simulink model "AeroTabularize"  (R2024b)
settings: Solver=VariableStepAuto  StartTime=0.0  StopTime=20  RelTol=1e-3
undefined symbols (not defined in the file or in its folder): uavParam
libraries: sharedutil x4, aerolibadyn x3, aerolibtransform2 x2, matrix_library x1, aerolibatmos2 x1, aerolibutil x1
(part 1 of 2)
settings Model: Creator=mhcho  LastModifiedBy=mhcho

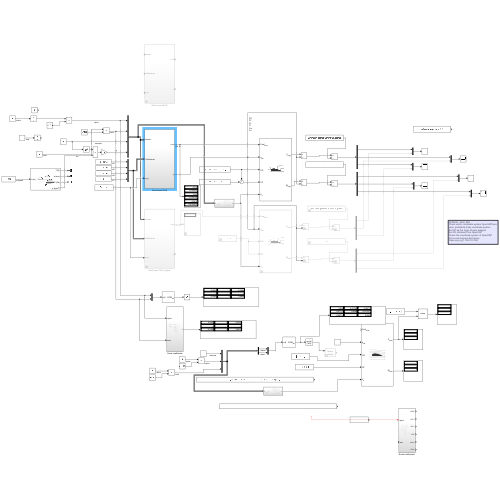
[thumbnail: Simulink's stored preview of the top-level diagram]
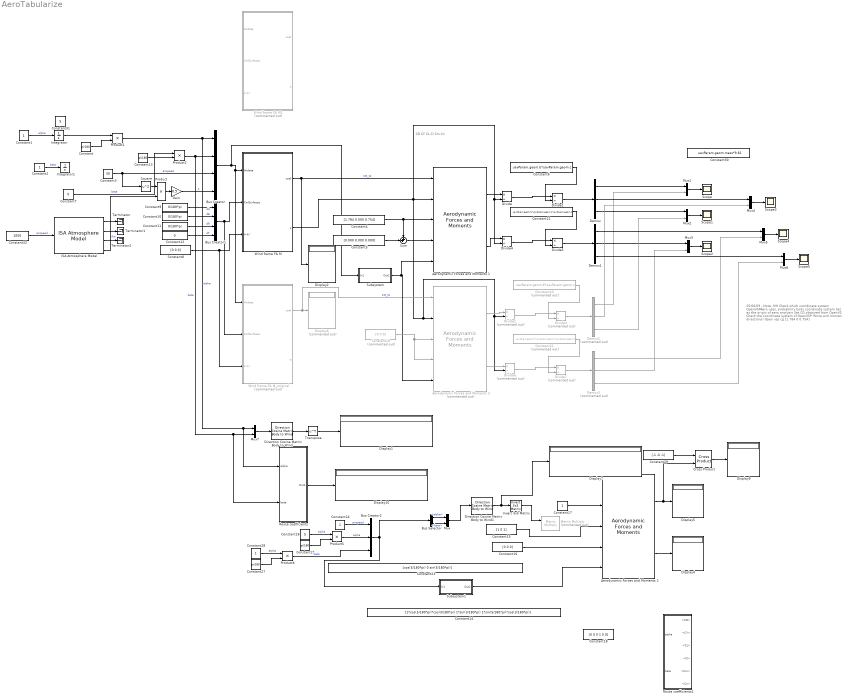
== system AeroTabularize ==
  note: CD
      | CY
      | CL
      | Cl
      | Cm
      | Cn
  note: 25/06/09 - Note, MH
      | Check which coordinate system OpenVSPAero
      | uses, probability body coordinate system
      | Set CP as the origin of aero analysis
      | Set CG obtained from OpenVSP
      | Check the coordinate system of OpenVSP
      | (force and moment directions)
      | Open vsp cg [1.784 0 0.754]
  Aerodynamic Forces and Moments 1 : aerolibadyn/Aerodynamic Forces and Moments   inputAxes=Wind  outputForceAxes=Body  outputMomentAxes=Body  S=uavParam.geom.b*uavParam.geom.c  b=uavParam.geom.b  cbar=uavParam.geom.c
  Aerodynamic Forces and Moments 2 : aerolibadyn/Aerodynamic Forces and Moments   inputAxes=Wind  outputForceAxes=Body  outputMomentAxes=Body  S=1  b=1  cbar=1
  Aerodynamic Forces and Moments 3 : aerolibadyn/Aerodynamic Forces and Moments   Commented=on  inputAxes=Wind  outputForceAxes=Body  outputMomentAxes=Body  S=uavParam.geom.b*uavParam.geom.c  b=uavParam.geom.b  cbar=uavParam.geom.c
  Bus Creator : BusCreator  Inputs=4
  Bus Creator1 : BusCreator  Inputs=4
  Bus Creator2 : BusCreator  Inputs=3
  Bus Selector : BusSelector  OutputSignals=alpha,beta
  Constant{,13,25,27} (4 alike) : Constant  Value=pi/180
  Constant{1..2,17,24,28} (5 alike) : Constant
  Constant10 : Constant  Value=0/180*pi
  Constant11 : Constant  Value=0/180*pi
  Constant12 : Constant  Value=0
  Constant14 : Constant  Value=[1*cos(5/180*pi)*cos(3/180*pi) 1*sin(3/180*pi) 1*sin(5/180*pi)*cos(3/180*pi)]
  Constant15 : Constant  Value=[1 0 1]
  Constant16 : Constant  Value=[0 0 0]
  Constant18 : Constant  Value=[0 0 0 1 0 0]
  Constant19 : Constant  Commented=on  Value=[0 0 0]
  Constant20 : Constant  Commented=on  Value=uavParam.geom.b*uavParam.geom.c
  Constant21 : Constant  Value=uavParam.geom.b*uavParam.geom.c*uavParam.geom.c
  Constant22 : Constant  Commented=on  Value=uavParam.geom.b*uavParam.geom.c*uavParam.geom.c
  Constant23 : Constant  Value=[cos(5/180*pi) 0 sin(5/180*pi)]
  Constant26 : Constant  Value=5
  Constant29 : Constant  Value=[-1 -0 -1]
  Constant3 : Constant  Value=30
  Constant30 : Constant  Value=uavParam.geom.mass*9.81
  Constant31 : Constant  Value=5
  Constant32 : Constant  Value=1000
  Constant4 : Constant  Value=[1.784 0.000 0.754]
  Constant5 : Constant  Value=[0.000 0.000 0.000]
  Constant6 : Constant  Value=uavParam.geom.b*uavParam.geom.c
  Constant7 : Constant  Value=0
  Constant8 : Constant  Value=[0 0 0]
  Constant9 : Constant  Value=0/180*pi
  Cross Product : matrix_library/Cross Product
  Demux : Demux  Outputs=3
  Demux1 : Demux  Outputs=3
  Demux2 : Demux  Commented=on  Outputs=3
  Demux3 : Demux  Commented=on  Outputs=3
  Direction Cosine Matrix Body to Wind : aerolibtransform2/Direction Cosine Matrix Body to Wind
  Direction Cosine Matrix Body to Wind1 : aerolibtransform2/Direction Cosine Matrix Body to Wind
  Display{1..2,4..5,7,9..10} (7 alike) : Display
  Display6 : Display  Commented=on
  Divide{,1,4..5} (4 alike) : Product  Inputs=*/
  Divide{2..3,6..7} (4 alike) : Product  Commented=on  Inputs=*/
  Gain : Gain  Gain=0.5
  ISA Atmosphere Model : aerolibatmos2/ISA Atmosphere Model  useExtended=off  action=Warning  custom=off  viscosityOut=off  g=9.80665  gamma=1.4  R=287.0531  L=0.0065  h_trop=11000  h_strat=20000  rho0=1.225  P0=101325  T0=288.15  h0=0  S=110.4  Tref=273.15  muref=1.716e-5
  Integrator : Integrator  InitialCondition=-5
  Integrator1 : Integrator  InitialCondition=-10
  Invert 3x3 Matrix : aerolibutil/Invert  3x3 Matrix
  Matrix Multiply : Product  Commented=on  Multiplication=Matrix(*)
  Mux{,1..7} (8 alike) : Mux  Inputs=2
  Product{,1..2,5..6} (5 alike) : Product
  Route coefficients : Subsystem
  Route coefficients1 : Subsystem
  Scope{,1..5} (6 alike) : Scope
  Square : Math  Operator=square
  Subsystem : Subsystem
  Subsystem1 : Subsystem
  Sum : Sum  Inputs=++|
  Terminator : Terminator
  Terminator1 : Terminator
  Terminator2 : Terminator
  Transpose : Math  Operator=transpose  SignedPower=on
  Wind frame F& M : Subsystem
  Wind frame F& M1 : Subsystem  Commented=on
  Wind frame F& M_original : Subsystem  Commented=on
  wires:
  Bus Creator/1 -> Subsystem/1(In1), Wind frame F& M_original/1(Airdata), Wind frame F& M/1(Airdata)
  Wind frame F& M/1(coef) -> Display2/1, Aerodynamic Forces and Moments 1/1  "FM_W"
  Wind frame F& M/2(q) -> Divide6/2, Divide2/2, Aerodynamic Forces and Moments 3/2, Aerodynamic Forces and Moments 1/2, Divide4/2, Divide/2
  Constant3/1 -> Square/1, Bus Creator/3  "airspeed"
  Gain/1 -> Bus Creator/4  "q"
  ISA Atmosphere Model/4 -> Product/2  "rho"
  Bus Creator1/1 -> Wind frame F& M_original/2(CtrlSurfaces), Wind frame F& M/2(CtrlSurfaces)
  Constant8/1 -> Wind frame F& M_original/3(p,q,r), Wind frame F& M/3(p,q,r)
  Square/1 -> Product/1
  Product/1 -> Gain/1
  Constant/1 -> Product1/2
  Constant13/1 -> Product2/2
  Product1/1 -> Route coefficients/1(alpha), Mux7/1, Bus Creator/1  "alpha"
  Product2/1 -> Route coefficients/2(beta), Mux7/2, Bus Creator/2  "beta"
  Constant16/1 -> Aerodynamic Forces and Moments 2/4
  Constant17/1 -> Aerodynamic Forces and Moments 2/2
  Aerodynamic Forces and Moments 2/2 -> Display4/1
  Aerodynamic Forces and Moments 2/1 -> Cross Product/2, Display5/1
  Wind frame F& M_original/1(coef) -> Aerodynamic Forces and Moments 3/1, Display6/1  "FM_W"
  Subsystem/1(Out1) -> Aerodynamic Forces and Moments 1/5, Aerodynamic Forces and Moments 3/5
  Constant9/1 -> Bus Creator1/1  "dA"
  Constant10/1 -> Bus Creator1/2  "dE"
  Constant11/1 -> Bus Creator1/3  "dR"
  Constant12/1 -> Bus Creator1/4  "dT"
  Aerodynamic Forces and Moments 1/1 -> Divide/1
  Divide1/1 -> Demux/1
  Divide/1 -> Divide1/1
  Constant6/1 -> Divide1/2
  Constant19/1 -> Aerodynamic Forces and Moments 3/4, Aerodynamic Forces and Moments 3/3
  Divide3/1 -> Demux2/1
  Divide2/1 -> Divide3/1
  Constant20/1 -> Divide3/2
  Aerodynamic Forces and Moments 3/1 -> Divide2/1
  Divide5/1 -> Demux1/1
  Divide4/1 -> Divide5/1
  Constant21/1 -> Divide5/2
  Aerodynamic Forces and Moments 1/2 -> Divide4/1
  Constant22/1 -> Divide7/2
  Divide7/1 -> Demux3/1
  Divide6/1 -> Divide7/1
  Aerodynamic Forces and Moments 3/2 -> Divide6/1
  Direction Cosine Matrix Body to Wind1/1 -> Display7/1, Invert 3x3 Matrix/1
  Invert 3x3 Matrix/1 -> Matrix Multiply/1
  Constant25/1 -> Product5/2
  Constant26/1 -> Product5/1  "alpha"
  Product5/1 -> Bus Creator2/2  "alpha"
  Constant27/1 -> Product6/2
  Constant28/1 -> Product6/1  "alpha"
  Product6/1 -> Bus Creator2/3  "beta"
  Constant24/1 -> Bus Creator2/1  "airspeed"
  Bus Creator2/1 -> Subsystem1/1(In1), Bus Selector/1
  Subsystem1/1(Out1) -> Aerodynamic Forces and Moments 2/5
  Bus Selector/1 -> Mux/1  "<alpha>"
  Bus Selector/2 -> Mux/2  "<beta>"
  Mux/1 -> Direction Cosine Matrix Body to Wind1/1
  Constant15/1 -> Aerodynamic Forces and Moments 2/3
  Constant29/1 -> Cross Product/1
  Cross Product/1 -> Display9/1
  Route coefficients/1(Out1) -> Display10/1
  ? -> Route coefficients1/1(alpha)
  Constant4/1 -> Sum/1, Aerodynamic Forces and Moments 1/3
  Sum/1 -> Aerodynamic Forces and Moments 1/4
  Constant5/1 -> Sum/2
  Constant1/1 -> Integrator/1  "alpha"
  Demux/1 -> Mux1/1
  Demux2/1 -> Mux1/2
  Demux/3 -> Mux2/1
  Demux1/2 -> Mux3/1
  Demux3/2 -> Mux3/2
  Mux2/1 -> Scope1/1
  Mux3/1 -> Scope2/1
  Mux1/1 -> Scope/1
  Demux2/3 -> Mux2/2
  Mux4/1 -> Scope3/1
  Demux/2 -> Mux4/1
  Demux2/2 -> Mux4/2
  Mux5/1 -> Scope4/1
  Demux1/1 -> Mux5/1
  Demux3/1 -> Mux5/2
  Mux6/1 -> Scope5/1
  Demux1/3 -> Mux6/1
  Demux3/3 -> Mux6/2
  Constant2/1 -> Integrator1/1  "beta"
  Direction Cosine Matrix Body to Wind/1 -> Transpose/1
  Mux7/1 -> Direction Cosine Matrix Body to Wind/1
  Transpose/1 -> Display1/1
  Constant32/1 -> ISA Atmosphere Model/1  "airspeed"
  ISA Atmosphere Model/1 -> Terminator/1
  ISA Atmosphere Model/2 -> Terminator1/1
  ISA Atmosphere Model/3 -> Terminator2/1
  Constant7/1 -> Product2/1  "beta"
  Integrator/1 -> Product1/1

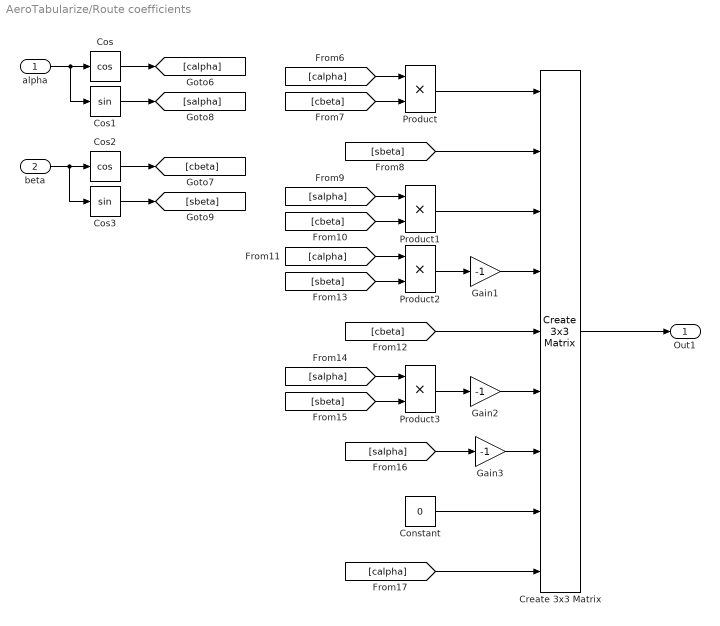
== system AeroTabularize/Route coefficients ==
  alpha : Inport
  beta : Inport  Port=2
  Constant : Constant  Value=0
  Cos : Trigonometry  Operator=cos
  Cos1 : Trigonometry
  Cos2 : Trigonometry  Operator=cos
  Cos3 : Trigonometry
  Create 3x3 Matrix : sharedutil/Create 3x3 Matrix  aMode=aMode
  Gain1 : Gain  Gain=-1
  Gain2 : Gain  Gain=-1
  Gain3 : Gain  Gain=-1
  Product{,1..3} (4 alike) : Product
  Out1 : Outport
  wires:
  Cos/1 -> [calpha]
  alpha/1 -> Cos1/1, Cos/1
  Cos1/1 -> [salpha]
  Cos2/1 -> [cbeta]
  Cos3/1 -> [sbeta]
  beta/1 -> Cos3/1, Cos2/1
  [calpha] -> Product/1
  [cbeta] -> Product/2
  Product/1 -> Create 3x3 Matrix/1
  [sbeta] -> Create 3x3 Matrix/2
  Product1/1 -> Create 3x3 Matrix/3
  [salpha] -> Product1/1
  [cbeta] -> Product1/2
  [calpha] -> Product2/1
  Product2/1 -> Gain1/1
  [sbeta] -> Product2/2
  Gain1/1 -> Create 3x3 Matrix/4
  [cbeta] -> Create 3x3 Matrix/5
  Product3/1 -> Gain2/1
  [salpha] -> Product3/1
  [sbeta] -> Product3/2
  Gain2/1 -> Create 3x3 Matrix/6
  Gain3/1 -> Create 3x3 Matrix/7
  [salpha] -> Gain3/1
  Constant/1 -> Create 3x3 Matrix/8
  [calpha] -> Create 3x3 Matrix/9
  Create 3x3 Matrix/1 -> Out1/1

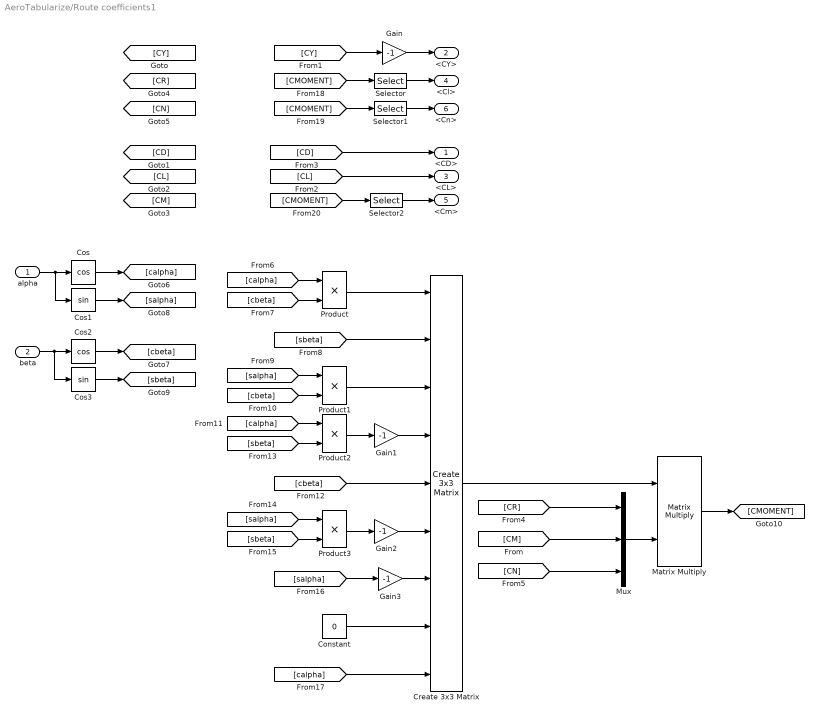
== system AeroTabularize/Route coefficients1 ==
  alpha : Inport
  beta : Inport  Port=2
  Constant : Constant  Value=0
  Cos : Trigonometry  Operator=cos
  Cos1 : Trigonometry
  Cos2 : Trigonometry  Operator=cos
  Cos3 : Trigonometry
  Create 3x3 Matrix : sharedutil/Create 3x3 Matrix  aMode=aMode
  Gain{,1..3} (4 alike) : Gain  Gain=-1
  Matrix Multiply : Product  Multiplication=Matrix(*)
  Mux : Mux  Inputs=3
  Product{,1..3} (4 alike) : Product
  Selector : Selector  InputPortWidth=3  IndexOptions=Index vector (dialog)  Indices=[1]  OutputSizes=1
  Selector1 : Selector  InputPortWidth=3  IndexOptions=Index vector (dialog)  Indices=[3]  OutputSizes=1
  Selector2 : Selector  InputPortWidth=3  IndexOptions=Index vector (dialog)  Indices=[2]  OutputSizes=1
  <CD> : Outport
  <CY> : Outport  Port=2
  <CL> : Outport  Port=3
  <Cl> : Outport  Port=4
  <Cm> : Outport  Port=5
  <Cn> : Outport  Port=6
  wires:
  ? -> [CY]
  [CY] -> Gain/1
  ? -> [CD]
  ? -> [CL]
  [CL] -> <CL>/1
  [CD] -> <CD>/1
  ? -> [CM]
  ? -> [CR]
  ? -> [CN]
  Gain/1 -> <CY>/1
  Cos/1 -> [calpha]
  alpha/1 -> Cos1/1, Cos/1
  Cos1/1 -> [salpha]
  Cos2/1 -> [cbeta]
  Cos3/1 -> [sbeta]
  beta/1 -> Cos3/1, Cos2/1
  [calpha] -> Product/1
  [cbeta] -> Product/2
  Product/1 -> Create 3x3 Matrix/1
  [sbeta] -> Create 3x3 Matrix/2
  Product1/1 -> Create 3x3 Matrix/3
  [salpha] -> Product1/1
  [cbeta] -> Product1/2
  [calpha] -> Product2/1
  Product2/1 -> Gain1/1
  [sbeta] -> Product2/2
  Gain1/1 -> Create 3x3 Matrix/4
  [cbeta] -> Create 3x3 Matrix/5
  Product3/1 -> Gain2/1
  [salpha] -> Product3/1
  [sbeta] -> Product3/2
  Gain2/1 -> Create 3x3 Matrix/6
  Gain3/1 -> Create 3x3 Matrix/7
  [salpha] -> Gain3/1
  Constant/1 -> Create 3x3 Matrix/8
  [calpha] -> Create 3x3 Matrix/9
  Create 3x3 Matrix/1 -> Matrix Multiply/1
  Mux/1 -> Matrix Multiply/2
  [CM] -> Mux/2
  [CR] -> Mux/1
  [CN] -> Mux/3
  Matrix Multiply/1 -> [CMOMENT]
  Selector/1 -> <Cl>/1
  [CMOMENT] -> Selector/1
  Selector1/1 -> <Cn>/1
  [CMOMENT] -> Selector1/1
  [CMOMENT] -> Selector2/1
  Selector2/1 -> <Cm>/1

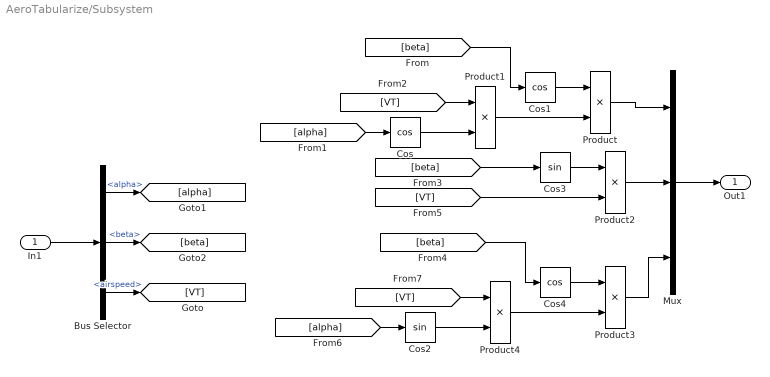
== system AeroTabularize/Subsystem ==
  In1 : Inport
  Bus Selector : BusSelector  OutputSignals=alpha,beta,airspeed
  Cos : Trigonometry  Operator=cos
  Cos1 : Trigonometry  Operator=cos
  Cos2 : Trigonometry
  Cos3 : Trigonometry
  Cos4 : Trigonometry  Operator=cos
  Mux : Mux  Inputs=3
  Product{,1..4} (5 alike) : Product
  Out1 : Outport
  wires:
  In1/1 -> Bus Selector/1
  Bus Selector/3 -> [VT]  "<airspeed>"
  Bus Selector/1 -> [alpha]  "<alpha>"
  Bus Selector/2 -> [beta]  "<beta>"
  Mux/1 -> Out1/1
  Product/1 -> Mux/1
  Product1/1 -> Product/2
  Cos/1 -> Product1/2
  Cos1/1 -> Product/1
  [alpha] -> Cos/1
  [VT] -> Product1/1
  [beta] -> Cos1/1
  Cos3/1 -> Product2/1
  [beta] -> Cos3/1
  [VT] -> Product2/2
  Product2/1 -> Mux/2
  Cos4/1 -> Product3/1
  [VT] -> Product4/1
  [alpha] -> Cos2/1
  [beta] -> Cos4/1
  Product4/1 -> Product3/2
  Cos2/1 -> Product4/2
  Product3/1 -> Mux/3

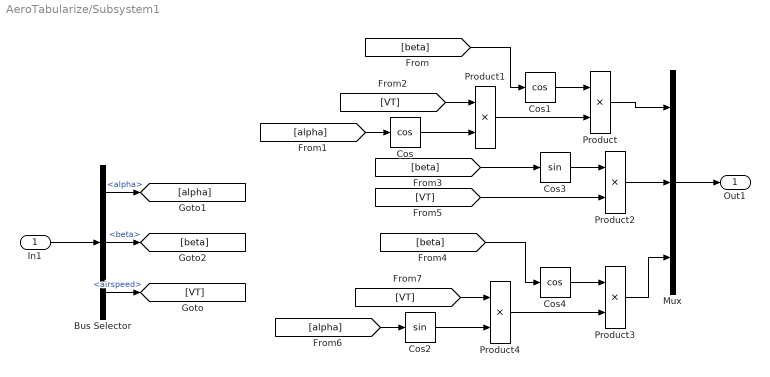
== system AeroTabularize/Subsystem1 ==
  In1 : Inport
  Bus Selector : BusSelector  OutputSignals=alpha,beta,airspeed
  Cos : Trigonometry  Operator=cos
  Cos1 : Trigonometry  Operator=cos
  Cos2 : Trigonometry
  Cos3 : Trigonometry
  Cos4 : Trigonometry  Operator=cos
  Mux : Mux  Inputs=3
  Product{,1..4} (5 alike) : Product
  Out1 : Outport
  wires:
  In1/1 -> Bus Selector/1
  Bus Selector/3 -> [VT]  "<airspeed>"
  Bus Selector/1 -> [alpha]  "<alpha>"
  Bus Selector/2 -> [beta]  "<beta>"
  Mux/1 -> Out1/1
  Product/1 -> Mux/1
  Product1/1 -> Product/2
  Cos/1 -> Product1/2
  Cos1/1 -> Product/1
  [alpha] -> Cos/1
  [VT] -> Product1/1
  [beta] -> Cos1/1
  Cos3/1 -> Product2/1
  [beta] -> Cos3/1
  [VT] -> Product2/2
  Product2/1 -> Mux/2
  Cos4/1 -> Product3/1
  [VT] -> Product4/1
  [alpha] -> Cos2/1
  [beta] -> Cos4/1
  Product4/1 -> Product3/2
  Cos2/1 -> Product4/2
  Product3/1 -> Mux/3

== system AeroTabularize/Wind frame F& M ==
  Airdata : Inport
  CtrlSurfaces : Inport  Port=2
  p,q,r : Inport  Port=3
  Bus Selector : BusSelector  OutputSignals=q
  Bus Selector1 : BusSelector  OutputSignals=dA,dR
  Bus Selector2 : BusSelector  OutputSignals=dE
  Bus Selector3 : BusSelector  OutputSignals=dA,dR
  Bus Selector4 : BusSelector  OutputSignals=alpha,beta
  Bus Selector6 : BusSelector  OutputSignals=alpha,beta,airspeed
  Bus Selector7 : BusSelector  OutputSignals=alpha,airspeed
  Lateral Channel : Subsystem
  Longitudinal Channel : Subsystem
  Mux : Mux  Inputs=6
  Route coefficients : Subsystem
  coef : Outport  PortDimensions=6  VectorParamsAs1DForOutWhenUnconnected=off
  q : Outport  Port=2
  wires:
  Bus Selector7/2 -> Longitudinal Channel/2(Airpseed)  "<airspeed>"
  Bus Selector7/1 -> Longitudinal Channel/1(alpha)  "<alpha>"
  Bus Selector6/3 -> Lateral Channel/3(Airspeed)  "<airspeed>"
  Bus Selector6/2 -> Lateral Channel/2(beta)  "<beta>"
  Airdata/1 -> Bus Selector7/1, Bus Selector6/1, Bus Selector4/1, Bus Selector/1
  Bus Selector2/1 -> Longitudinal Channel/3(dE)  "<dE>"
  Bus Selector1/2 -> Lateral Channel/5(dR)  "<dR>"
  Bus Selector1/1 -> Lateral Channel/4(dA)  "<dA>"
  CtrlSurfaces/1 -> Bus Selector3/1, Bus Selector2/1, Bus Selector1/1
  p,q,r/1 -> Lateral Channel/6(p,q,r), Longitudinal Channel/4(p,q,r)
  Mux/1 -> coef/1
  Longitudinal Channel/1(Longitudinal) -> Route coefficients/2(Longitudinal)
  Route coefficients/1(<CD>) -> Mux/1
  Route coefficients/2(<CC>) -> Mux/2
  Route coefficients/3(<CL>) -> Mux/3
  Route coefficients/4(<Cl>) -> Mux/4
  Route coefficients/5(<Cm>) -> Mux/5
  Route coefficients/6(<Cn>) -> Mux/6
  Bus Selector/1 -> q/1  "<q>"
  Bus Selector3/1 -> Longitudinal Channel/5(dA)  "<dA>"
  Bus Selector3/2 -> Longitudinal Channel/6(dR)  "<dR>"
  Lateral Channel/1(Lateral) -> Route coefficients/1(Lateral)
  Bus Selector4/1 -> Route coefficients/3(alpha)  "<alpha>"
  Bus Selector4/2 -> Route coefficients/4(beta)  "<beta>"
  Bus Selector6/1 -> Lateral Channel/1(alpha)  "<alpha>"

== system AeroTabularize/Wind frame F& M1 ==
  Airdata : Inport
  CtrlSurfaces : Inport  Port=2
  p,q,r : Inport  Port=3
  Bus Selector : BusSelector  OutputSignals=q
  Bus Selector1 : BusSelector  OutputSignals=dA,dR
  Bus Selector2 : BusSelector  OutputSignals=dE
  Bus Selector3 : BusSelector  OutputSignals=dA,dR
  Bus Selector4 : BusSelector  OutputSignals=alpha,beta
  Bus Selector6 : BusSelector  OutputSignals=beta,airspeed
  Bus Selector7 : BusSelector  OutputSignals=alpha,airspeed
  Lateral Channel : Subsystem
  Longitudinal Channel : Subsystem
  Mux : Mux  Inputs=6
  Route coefficients : Subsystem
  coef : Outport  PortDimensions=6  VectorParamsAs1DForOutWhenUnconnected=off
  q : Outport  Port=2
  wires:
  Bus Selector7/2 -> Longitudinal Channel/2(Airpseed)  "<airspeed>"
  Bus Selector7/1 -> Longitudinal Channel/1(alpha)  "<alpha>"
  Bus Selector6/2 -> Lateral Channel/2(Airspeed)  "<airspeed>"
  Bus Selector6/1 -> Lateral Channel/1(beta)  "<beta>"
  Airdata/1 -> Bus Selector4/1, Bus Selector/1, Bus Selector6/1, Bus Selector7/1
  Bus Selector2/1 -> Longitudinal Channel/3(dE)  "<dE>"
  Bus Selector1/2 -> Lateral Channel/4(dR)  "<dR>"
  Bus Selector1/1 -> Lateral Channel/3(dA)  "<dA>"
  CtrlSurfaces/1 -> Bus Selector1/1, Bus Selector3/1, Bus Selector2/1
  p,q,r/1 -> Lateral Channel/5(p,q,r), Longitudinal Channel/4(p,q,r)
  Mux/1 -> coef/1
  Longitudinal Channel/1(Longitudinal) -> Route coefficients/2(Longitudinal)
  Route coefficients/1(<CD>) -> Mux/1
  Route coefficients/2(<CY>) -> Mux/2
  Route coefficients/3(<CL>) -> Mux/3
  Route coefficients/4(<Cl>) -> Mux/4
  Route coefficients/5(<Cm>) -> Mux/5
  Route coefficients/6(<Cn>) -> Mux/6
  Bus Selector/1 -> q/1  "<q>"
  Bus Selector3/1 -> Longitudinal Channel/5(dA)  "<dA>"
  Bus Selector3/2 -> Longitudinal Channel/6(dR)  "<dR>"
  Lateral Channel/1(Lateral) -> Route coefficients/1(Lateral)
  Bus Selector4/1 -> Route coefficients/3(alpha)  "<alpha>"
  Bus Selector4/2 -> Route coefficients/4(beta)  "<beta>"

== system AeroTabularize/Wind frame F& M_original ==
  Airdata : Inport
  CtrlSurfaces : Inport  Port=2
  p,q,r : Inport  Port=3
  Bus Selector : BusSelector  OutputSignals=q
  Bus Selector1 : BusSelector  OutputSignals=dA,dR
  Bus Selector2 : BusSelector  OutputSignals=dE,dA,dR
  Bus Selector6 : BusSelector  OutputSignals=beta,airspeed
  Bus Selector7 : BusSelector  OutputSignals=alpha,airspeed
  Lateral Channel : Subsystem
  Longitudinal Channel : Subsystem
  Mux : Mux  Inputs=6
  Route coefficients : Subsystem
  coef : Outport  PortDimensions=6  VectorParamsAs1DForOutWhenUnconnected=off
  q : Outport  Port=2
  wires:
  Bus Selector7/2 -> Longitudinal Channel/2(Airpseed)  "<airspeed>"
  Bus Selector7/1 -> Longitudinal Channel/1(alpha)  "<alpha>"
  Bus Selector6/2 -> Lateral Channel/2(Airspeed)  "<airspeed>"
  Bus Selector6/1 -> Lateral Channel/1(beta)  "<beta>"
  Airdata/1 -> Bus Selector/1, Bus Selector6/1, Bus Selector7/1
  Bus Selector2/1 -> Longitudinal Channel/3(dE)  "<dE>"
  Bus Selector1/2 -> Lateral Channel/4(dR)  "<dR>"
  Bus Selector1/1 -> Lateral Channel/3(dA)  "<dA>"
  CtrlSurfaces/1 -> Bus Selector1/1, Bus Selector2/1
  p,q,r/1 -> Lateral Channel/5(p,q,r), Longitudinal Channel/4(p,q,r)
  Bus Selector2/2 -> Longitudinal Channel/5(dA)  "<dA>"
  Bus Selector2/3 -> Longitudinal Channel/6(dR)  "<dR>"
  Mux/1 -> coef/1
  Lateral Channel/1(Lateral) -> Route coefficients/1(Lateral)
  Longitudinal Channel/1(Longitudinal) -> Route coefficients/2(Longitudinal)
  Route coefficients/1(<CD>) -> Mux/1
  Route coefficients/2(<CY>) -> Mux/2
  Route coefficients/3(<CL>) -> Mux/3
  Route coefficients/4(<Cl>) -> Mux/4
  Route coefficients/5(<Cm>) -> Mux/5
  Route coefficients/6(<Cn>) -> Mux/6
  Bus Selector/1 -> q/1  "<q>"

== system AeroTabularize/Wind frame F& M/Lateral Channel ==
  alpha : Inport
  beta : Inport  Port=2
  Airspeed : Inport  Port=3
  dA : Inport  Port=4
  dR : Inport  Port=5
  p,q,r : Inport  Port=6
  Bus Creator : BusCreator  Inputs=3
  CY : Subsystem
  Cl : Subsystem
  Cn : Subsystem
  Lateral : Outport  VectorParamsAs1DForOutWhenUnconnected=off
  wires:
  p,q,r/1 -> CY/4(p,q,r), Cl/5(p,q,r), Cn/5(p,q,r)
  Airspeed/1 -> CY/5(Airspeed), Cl/6(Airspeed), Cn/6(Airspeed)
  dR/1 -> CY/3(dR), Cl/4(dR), Cn/4(dR)
  dA/1 -> Cn/3(dA), Cl/3(dA)
  beta/1 -> CY/2(beta), Cn/2(beta), Cl/2(beta)
  Bus Creator/1 -> Lateral/1
  CY/1(CS) -> Bus Creator/1  "CS"
  alpha/1 -> Cn/1(alpha), Cl/1(alpha), CY/1(alpha)
  Cl/1(Cl) -> Bus Creator/2  "Cl"
  Cn/1(Cn) -> Bus Creator/3  "Cn"

== system AeroTabularize/Wind frame F& M/Longitudinal Channel ==
  alpha : Inport
  Airpseed : Inport  Port=2
  dE : Inport  Port=3
  p,q,r : Inport  Port=4
  dA : Inport  Port=5
  dR : Inport  Port=6
  Bus Creator : BusCreator  Inputs=3
  CD : Subsystem
  CL : Subsystem
  Cm : Subsystem
  Saturation : Saturate  UpperLimit=max(uavParam.aero.alpha_lon)  LowerLimit=min(uavParam.aero.alpha_lon)  LinearizeAsGain=off  ZeroCross=off
  Transfer Fcn : TransferFcn  Numerator=[1 0]  Denominator=[0.1 1]
  Longitudinal : Outport  VectorParamsAs1DForOutWhenUnconnected=off
  wires:
  Transfer Fcn/1 -> CL/2(alpha_dot)
  Airpseed/1 -> CL/5(Airspeed), Cm/4(Airspeed)
  p,q,r/1 -> CL/4(p,q,r), Cm/3(p,q,r)
  Bus Creator/1 -> Longitudinal/1
  dE/1 -> Cm/2(dE), CD/4(dE), CL/3(dE)
  CD/1(CD) -> Bus Creator/1  "CD"
  alpha/1 -> Saturation/1
  dR/1 -> CD/3(dR)
  dA/1 -> CD/2(dA), CL/6(dA)
  Saturation/1 -> CD/1(alpha), CL/1(alpha), Cm/1(alpha), Transfer Fcn/1
  Cm/1(Cm) -> Bus Creator/3  "Cm"
  CL/1(CL) -> Bus Creator/2  "CL"

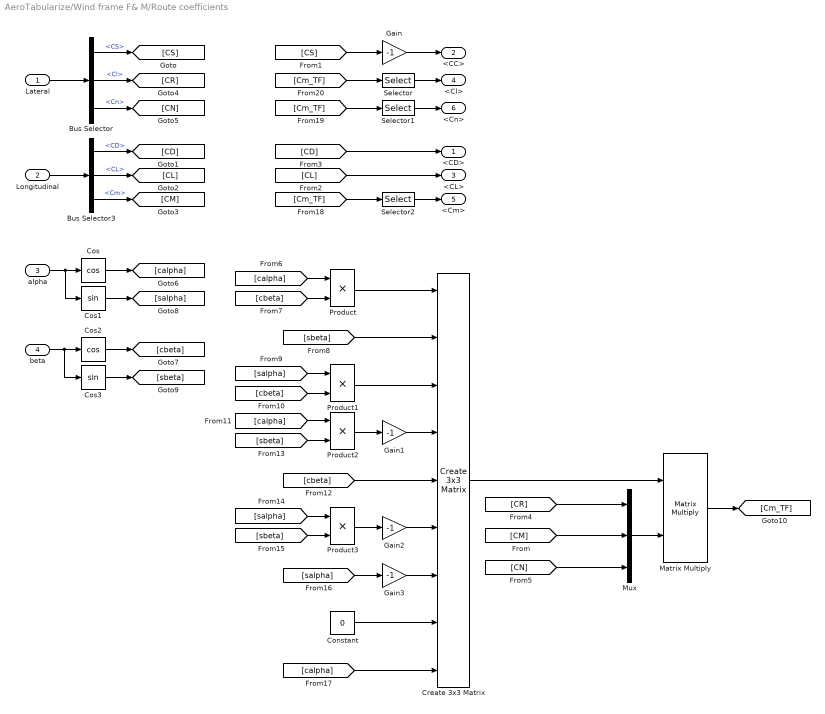
== system AeroTabularize/Wind frame F& M/Route coefficients ==
  Lateral : Inport
  Longitudinal : Inport  Port=2
  alpha : Inport  Port=3
  beta : Inport  Port=4
  Bus Selector : BusSelector  OutputSignals=CS,Cl,Cn
  Bus Selector3 : BusSelector  OutputSignals=CD,CL,Cm
  Constant : Constant  Value=0
  Cos : Trigonometry  Operator=cos
  Cos1 : Trigonometry
  Cos2 : Trigonometry  Operator=cos
  Cos3 : Trigonometry
  Create 3x3 Matrix : sharedutil/Create 3x3 Matrix  aMode=aMode
      settings: LibrarySourceBlock=aerolibutil/Create 3x3 Matrix
  Gain{,1..3} (4 alike) : Gain  Gain=-1
  Matrix Multiply : Product  Multiplication=Matrix(*)
  Mux : Mux  Inputs=3
  Product{,1..3} (4 alike) : Product
  Selector : Selector  InputPortWidth=3  IndexOptions=Index vector (dialog)  Indices=[1]  OutputSizes=1
  Selector1 : Selector  InputPortWidth=3  IndexOptions=Index vector (dialog)  Indices=[3]  OutputSizes=1
  Selector2 : Selector  InputPortWidth=3  IndexOptions=Index vector (dialog)  Indices=[2]  OutputSizes=1
  <CD> : Outport
  <CC> : Outport  Port=2
  <CL> : Outport  Port=3
  <Cl> : Outport  Port=4
  <Cm> : Outport  Port=5
  <Cn> : Outport  Port=6
  wires:
  Lateral/1 -> Bus Selector/1
  Longitudinal/1 -> Bus Selector3/1
  Bus Selector/1 -> [CS]  "<CS>"
  Bus Selector3/1 -> [CD]  "<CD>"
  Bus Selector3/2 -> [CL]  "<CL>"
  [CL] -> <CL>/1
  [CD] -> <CD>/1
  Bus Selector3/3 -> [CM]  "<Cm>"
  Bus Selector/2 -> [CR]  "<Cl>"
  Bus Selector/3 -> [CN]  "<Cn>"
  Cos/1 -> [calpha]
  alpha/1 -> Cos1/1, Cos/1
  Cos1/1 -> [salpha]
  Cos2/1 -> [cbeta]
  Cos3/1 -> [sbeta]
  beta/1 -> Cos3/1, Cos2/1
  [calpha] -> Product/1
  [cbeta] -> Product/2
  Product/1 -> Create 3x3 Matrix/1
  [sbeta] -> Create 3x3 Matrix/2
  Product1/1 -> Create 3x3 Matrix/3
  [salpha] -> Product1/1
  [cbeta] -> Product1/2
  [calpha] -> Product2/1
  Product2/1 -> Gain1/1
  [sbeta] -> Product2/2
  Gain1/1 -> Create 3x3 Matrix/4
  [cbeta] -> Create 3x3 Matrix/5
  Product3/1 -> Gain2/1
  [salpha] -> Product3/1
  [sbeta] -> Product3/2
  Gain2/1 -> Create 3x3 Matrix/6
  Gain3/1 -> Create 3x3 Matrix/7
  [salpha] -> Gain3/1
  Constant/1 -> Create 3x3 Matrix/8
  [calpha] -> Create 3x3 Matrix/9
  Create 3x3 Matrix/1 -> Matrix Multiply/1
  Mux/1 -> Matrix Multiply/2
  [CM] -> Mux/2
  Matrix Multiply/1 -> [Cm_TF]
  [Cm_TF] -> Selector/1
  [Cm_TF] -> Selector1/1
  [Cm_TF] -> Selector2/1
  [CR] -> Mux/1
  [CN] -> Mux/3
  Gain/1 -> <CC>/1
  [CS] -> Gain/1
  Selector2/1 -> <Cm>/1
  Selector/1 -> <Cl>/1
  Selector1/1 -> <Cn>/1

== system AeroTabularize/Wind frame F& M1/Lateral Channel ==
  beta : Inport
  Airspeed : Inport  Port=2
  dA : Inport  Port=3
  dR : Inport  Port=4
  p,q,r : Inport  Port=5
  Bus Creator : BusCreator  Inputs=3
  CY : Subsystem
  Cl : Subsystem
  Cn : Subsystem
  Lateral : Outport  VectorParamsAs1DForOutWhenUnconnected=off
  wires:
  p,q,r/1 -> Cn/4(p,q,r), Cl/4(p,q,r), CY/3(p,q,r)
  Airspeed/1 -> Cn/5(Airspeed), Cl/5(Airspeed), CY/4(Airspeed)
  dR/1 -> Cn/3(dR), Cl/3(dR), CY/2(dR)
  dA/1 -> Cl/2(dA), Cn/2(dA)
  beta/1 -> CY/1(beta), Cl/1(beta), Cn/1(beta)
  Bus Creator/1 -> Lateral/1
  CY/1(CY) -> Bus Creator/1  "CY"
  Cl/1(Cl) -> Bus Creator/2  "Cl"
  Cn/1(Cn) -> Bus Creator/3  "Cn"

== system AeroTabularize/Wind frame F& M1/Longitudinal Channel ==
  alpha : Inport
  Airpseed : Inport  Port=2
  dE : Inport  Port=3
  p,q,r : Inport  Port=4
  dA : Inport  Port=5
  dR : Inport  Port=6
  Bus Creator : BusCreator  Inputs=3
  CD : Subsystem
  CL : Subsystem
  Cm : Subsystem
  Saturation : Saturate  UpperLimit=max(uavParam.aero.alpha)  LowerLimit=min(uavParam.aero.alpha)  LinearizeAsGain=off  ZeroCross=off
  Transfer Fcn : TransferFcn  Numerator=[1 0]  Denominator=[0.1 1]
  Longitudinal : Outport  VectorParamsAs1DForOutWhenUnconnected=off
  wires:
  Transfer Fcn/1 -> CL/2(alpha_dot)
  Airpseed/1 -> CL/5(Airspeed), Cm/4(Airspeed)
  p,q,r/1 -> CL/4(p,q,r), Cm/3(p,q,r)
  Bus Creator/1 -> Longitudinal/1
  dE/1 -> Cm/2(dE), CD/4(dE), CL/3(dE)
  CD/1(CD) -> Bus Creator/1  "CD"
  alpha/1 -> Saturation/1
  dR/1 -> CD/3(dR)
  dA/1 -> CD/2(dA), CL/6(dA)
  Saturation/1 -> CD/1(alpha), CL/1(alpha), Cm/1(alpha), Transfer Fcn/1
  Cm/1(Cm) -> Bus Creator/3  "Cm"
  CL/1(CL) -> Bus Creator/2  "CL"

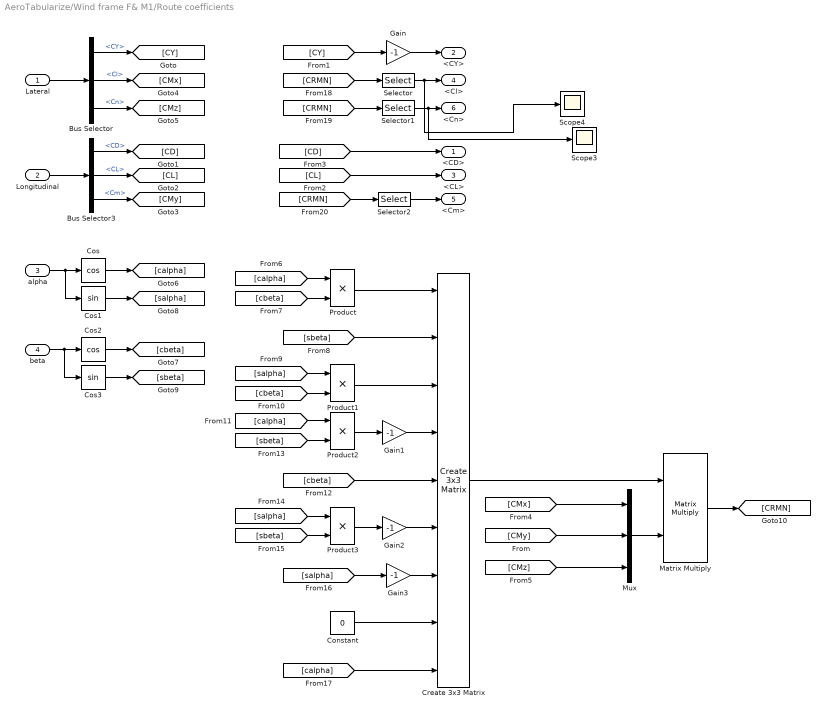
== system AeroTabularize/Wind frame F& M1/Route coefficients ==
  Lateral : Inport
  Longitudinal : Inport  Port=2
  alpha : Inport  Port=3
  beta : Inport  Port=4
  Bus Selector : BusSelector  OutputSignals=CY,Cl,Cn
  Bus Selector3 : BusSelector  OutputSignals=CD,CL,Cm
  Constant : Constant  Value=0
  Cos : Trigonometry  Operator=cos
  Cos1 : Trigonometry
  Cos2 : Trigonometry  Operator=cos
  Cos3 : Trigonometry
  Create 3x3 Matrix : sharedutil/Create 3x3 Matrix  aMode=aMode
      settings: LibrarySourceBlock=aerolibutil/Create 3x3 Matrix
  Gain{,1..3} (4 alike) : Gain  Gain=-1
  Matrix Multiply : Product  Multiplication=Matrix(*)
  Mux : Mux  Inputs=3
  Product{,1..3} (4 alike) : Product
  Scope3 : Scope
  Scope4 : Scope
  Selector : Selector  InputPortWidth=3  IndexOptions=Index vector (dialog)  Indices=[1]  OutputSizes=1
  Selector1 : Selector  InputPortWidth=3  IndexOptions=Index vector (dialog)  Indices=[3]  OutputSizes=1
  Selector2 : Selector  InputPortWidth=3  IndexOptions=Index vector (dialog)  Indices=[2]  OutputSizes=1
  <CD> : Outport
  <CY> : Outport  Port=2
  <CL> : Outport  Port=3
  <Cl> : Outport  Port=4
  <Cm> : Outport  Port=5
  <Cn> : Outport  Port=6
  wires:
  Lateral/1 -> Bus Selector/1
  Longitudinal/1 -> Bus Selector3/1
  Bus Selector/1 -> [CY]  "<CY>"
  Bus Selector3/1 -> [CD]  "<CD>"
  Bus Selector3/2 -> [CL]  "<CL>"
  [CL] -> <CL>/1
  [CD] -> <CD>/1
  Bus Selector3/3 -> [CMy]  "<Cm>"
  Bus Selector/2 -> [CMx]  "<Cl>"
  Bus Selector/3 -> [CMz]  "<Cn>"
  [CY] -> Gain/1
  Cos/1 -> [calpha]
  alpha/1 -> Cos1/1, Cos/1
  Cos1/1 -> [salpha]
  Cos2/1 -> [cbeta]
  Cos3/1 -> [sbeta]
  beta/1 -> Cos3/1, Cos2/1
  [calpha] -> Product/1
  [cbeta] -> Product/2
  Product/1 -> Create 3x3 Matrix/1
  [sbeta] -> Create 3x3 Matrix/2
  Product1/1 -> Create 3x3 Matrix/3
  [salpha] -> Product1/1
  [cbeta] -> Product1/2
  [calpha] -> Product2/1
  Product2/1 -> Gain1/1
  [sbeta] -> Product2/2
  Gain1/1 -> Create 3x3 Matrix/4
  [cbeta] -> Create 3x3 Matrix/5
  Product3/1 -> Gain2/1
  [salpha] -> Product3/1
  [sbeta] -> Product3/2
  Gain2/1 -> Create 3x3 Matrix/6
  Gain3/1 -> Create 3x3 Matrix/7
  [salpha] -> Gain3/1
  Constant/1 -> Create 3x3 Matrix/8
  [calpha] -> Create 3x3 Matrix/9
  Create 3x3 Matrix/1 -> Matrix Multiply/1
  Mux/1 -> Matrix Multiply/2
  [CMy] -> Mux/2
  Matrix Multiply/1 -> [CRMN]
  Selector/1 -> Scope4/1, <Cl>/1
  [CRMN] -> Selector/1
  Selector1/1 -> Scope3/1, <Cn>/1
  [CRMN] -> Selector1/1
  [CRMN] -> Selector2/1
  Selector2/1 -> <Cm>/1
  [CMx] -> Mux/1
  [CMz] -> Mux/3
  Gain/1 -> <CY>/1

== system AeroTabularize/Wind frame F& M_original/Lateral Channel ==
  beta : Inport
  Airspeed : Inport  Port=2
  dA : Inport  Port=3
  dR : Inport  Port=4
  p,q,r : Inport  Port=5
  Bus Creator : BusCreator  Inputs=3
  CY : Subsystem
  Cl : Subsystem
  Cn : Subsystem
  Lateral : Outport  VectorParamsAs1DForOutWhenUnconnected=off
  wires:
  Cl/1(Cl) -> Bus Creator/2  "Cl"
  p,q,r/1 -> CY/3(p,q,r), Cn/4(p,q,r), Cl/4(p,q,r)
  Airspeed/1 -> CY/4(Airspeed), Cn/5(Airspeed), Cl/5(Airspeed)
  dR/1 -> CY/2(dR), Cl/3(dR), Cn/3(dR)
  dA/1 -> Cl/2(dA), Cn/2(dA)
  beta/1 -> CY/1(beta), Cl/1(beta), Cn/1(beta)
  Cn/1(Cn) -> Bus Creator/3  "Cn"
  CY/1(CY) -> Bus Creator/1  "CY"
  Bus Creator/1 -> Lateral/1

== system AeroTabularize/Wind frame F& M_original/Longitudinal Channel ==
  alpha : Inport
  Airpseed : Inport  Port=2
  dE : Inport  Port=3
  p,q,r : Inport  Port=4
  dA : Inport  Port=5
  dR : Inport  Port=6
  Bus Creator : BusCreator  Inputs=3
  CD : Subsystem
  CL : Subsystem
  Cm : Subsystem
  Constant : Constant
  Saturation : Saturate  UpperLimit=14*pi/180  LowerLimit=-14*pi/180  LinearizeAsGain=off  ZeroCross=off
  Y-down : Gain  SaturateOnIntegerOverflow=on  OutDataTypeStr=Inherit: Same as input  ParamDataTypeStr=Inherit: Same as input
      settings: AttributesFormatString=%<Gain>
  Longitudinal : Outport  VectorParamsAs1DForOutWhenUnconnected=off
  wires:
  Airpseed/1 -> Cm/4(Airspeed), CL/5(Airspeed)
  p,q,r/1 -> Cm/3(p,q,r), CL/4(p,q,r)
  Bus Creator/1 -> Longitudinal/1
  Cm/1(Cm) -> Bus Creator/3  "Cm"
  CL/1(CL) -> CD/1(CL), Y-down/1
  dE/1 -> Cm/2(De), CD/4(dE), CL/3(dE)
  Y-down/1 -> Bus Creator/2  "CL"
  CD/1(CD) -> Bus Creator/1  "CD"
  alpha/1 -> Saturation/1
  dR/1 -> CD/3(dR)
  dA/1 -> CD/2(dA), CL/6(dA)
  Saturation/1 -> Cm/1(alpha), CL/1(alpha)
  Constant/1 -> CL/2(alpha_dot)

== system AeroTabularize/Wind frame F& M_original/Route coefficients ==
  Lateral : Inport
  Longitudinal : Inport  Port=2
  Bus Selector : BusSelector  OutputSignals=CY,Cl,Cn
  Bus Selector3 : BusSelector  OutputSignals=CD,CL,Cm
  <CD> : Outport
  <CY> : Outport  Port=2
  <CL> : Outport  Port=3
  <Cl> : Outport  Port=4
  <Cm> : Outport  Port=5
  <Cn> : Outport  Port=6
  wires:
  Bus Selector3/2 -> <CL>/1  "<CL>"
  Bus Selector/3 -> <Cn>/1  "<Cn>"
  Bus Selector/2 -> <Cl>/1  "<Cl>"
  Lateral/1 -> Bus Selector/1
  Bus Selector3/3 -> <Cm>/1  "<Cm>"
  Bus Selector3/1 -> <CD>/1  "<CD>"
  Longitudinal/1 -> Bus Selector3/1
  Bus Selector/1 -> <CY>/1  "<CY>"

== system AeroTabularize/Wind frame F& M/Lateral Channel/CY ==
  alpha : Inport
  beta : Inport  Port=2
  dR : Inport  Port=3
  p,q,r : Inport  Port=4
  Airspeed : Inport  Port=5
  1-D Lookup Table : Lookup_n-D  BreakpointsForDimension1=uavParam.aero.alpha_latdir  BreakpointsForDimension2=uavParam.aero.beta_latdir  Table=uavParam.aero.CS  ExtrapMethod=Clip  UseLastTableValue=on  InternalRulePriority=Speed  RndMeth=Simplest
      settings: InputPortMap=u0,u1
  Abs : Abs  Commented=on  SaturateOnIntegerOverflow=off
  CYDr : Constant  Value=uavParam.aero.CYDr
      settings: AttributesFormatString=%<Value>
  CYb : Constant  Commented=on  Value=uavParam.aero.CYb
      settings: AttributesFormatString=%<Value>
  Product : Product  Commented=on  SaturateOnIntegerOverflow=on  OutDataTypeStr=Inherit: Same as first input
  Product1 : Product  SaturateOnIntegerOverflow=on  OutDataTypeStr=Inherit: Same as first input
  Product2 : Product  Commented=on
  Sign : Signum  Commented=on
  Sum2 : Sum  Inputs=++++  SaturateOnIntegerOverflow=on
  roll factors : Subsystem
  CS : Outport  VectorParamsAs1DForOutWhenUnconnected=off
  wires:
  dR/1 -> Product1/2
  CYDr/1 -> Product1/1
  CYb/1 -> Product/1
  Airspeed/1 -> roll factors/2(Airspeed)
  p,q,r/1 -> roll factors/1(p,q,r)
  Sum2/1 -> CS/1
  beta/1 -> 1-D Lookup Table/2
  1-D Lookup Table/1 -> Sum2/1
  alpha/1 -> 1-D Lookup Table/1
  Sign/1 -> Product2/2
  Product1/1 -> Sum2/2
  roll factors/1(CSp) -> Sum2/3
  roll factors/2(CSr) -> Sum2/4

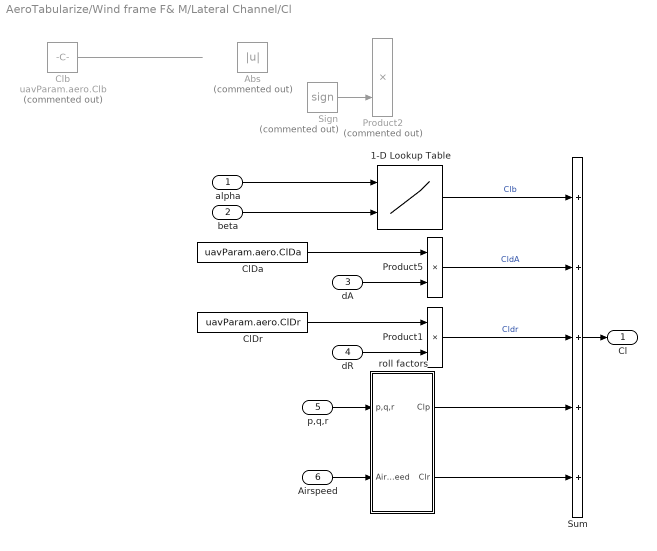
== system AeroTabularize/Wind frame F& M/Lateral Channel/Cl ==
  alpha : Inport
  beta : Inport  Port=2
  dA : Inport  Port=3
  dR : Inport  Port=4
  p,q,r : Inport  Port=5
  Airspeed : Inport  Port=6
  1-D Lookup Table : Lookup_n-D  BreakpointsForDimension1=uavParam.aero.alpha_latdir  BreakpointsForDimension2=uavParam.aero.beta_latdir  Table=uavParam.aero.CR  InternalRulePriority=Speed  RndMeth=Simplest
      settings: InputPortMap=u0,u1
  Abs : Abs  Commented=on  SaturateOnIntegerOverflow=off
  ClDa : Constant  Value=uavParam.aero.ClDa
      settings: AttributesFormatString=%<Value>
  ClDr : Constant  Value=uavParam.aero.ClDr
      settings: AttributesFormatString=%<Value>
  Clb : Constant  Commented=on  Value=uavParam.aero.Clb
      settings: AttributesFormatString=%<Value>
  Product1 : Product  SaturateOnIntegerOverflow=on  OutDataTypeStr=Inherit: Same as first input
  Product2 : Product  Commented=on
  Product5 : Product  SaturateOnIntegerOverflow=on  OutDataTypeStr=Inherit: Same as first input
  Sign : Signum  Commented=on
  Sum : Sum  Inputs=+++++  SaturateOnIntegerOverflow=on
  roll factors : Subsystem
  Cl : Outport  VectorParamsAs1DForOutWhenUnconnected=off
  wires:
  roll factors/1(Clp) -> Sum/4
  Product5/1 -> Sum/2  "CldA"
  Airspeed/1 -> roll factors/2(Airspeed)
  p,q,r/1 -> roll factors/1(p,q,r)
  roll factors/2(Clr) -> Sum/5
  Product1/1 -> Sum/3  "Cldr"
  Sum/1 -> Cl/1
  dR/1 -> Product1/2
  ClDr/1 -> Product1/1
  dA/1 -> Product5/2
  ClDa/1 -> Product5/1
  Clb/1 -> ?
  beta/1 -> 1-D Lookup Table/2
  Sign/1 -> Product2/2
  alpha/1 -> 1-D Lookup Table/1
  1-D Lookup Table/1 -> Sum/1  "Clb"

== system AeroTabularize/Wind frame F& M/Lateral Channel/Cn ==
  alpha : Inport
  beta : Inport  Port=2
  dA : Inport  Port=3
  dR : Inport  Port=4
  p,q,r : Inport  Port=5
  Airspeed : Inport  Port=6
  1-D Lookup Table : Lookup_n-D  BreakpointsForDimension1=uavParam.aero.alpha_latdir  BreakpointsForDimension2=uavParam.aero.beta_latdir  Table=uavParam.aero.CN  ExtrapMethod=Clip  UseLastTableValue=on  InternalRulePriority=Speed  RndMeth=Simplest
      settings: InputPortMap=u0,u1
  Abs : Abs  Commented=on  SaturateOnIntegerOverflow=off
  CnDa : Constant  Value=uavParam.aero.CnDa
      settings: AttributesFormatString=%<Value>
  CnDr : Constant  Value=uavParam.aero.CnDr
      settings: AttributesFormatString=%<Value>
  Cnb : Constant  Commented=on  Value=uavParam.aero.Cnb
      settings: AttributesFormatString=%<Value>
  Product1 : Product  SaturateOnIntegerOverflow=on  OutDataTypeStr=Inherit: Same as first input
  Product2 : Product  Commented=on
  Product5 : Product  SaturateOnIntegerOverflow=on  OutDataTypeStr=Inherit: Same as first input
  Sign : Signum  Commented=on
  Sum : Sum  Inputs=+++++  SaturateOnIntegerOverflow=on
  yaw factors : Subsystem
  Cn : Outport  VectorParamsAs1DForOutWhenUnconnected=off
  wires:
  Airspeed/1 -> yaw factors/2(Airspeed)
  p,q,r/1 -> yaw factors/1(p,q,r)
  CnDa/1 -> Product5/1
  Product5/1 -> Sum/2
  dA/1 -> Product5/2
  CnDr/1 -> Product1/1
  dR/1 -> Product1/2
  Sum/1 -> Cn/1
  Product1/1 -> Sum/3
  yaw factors/2(Cnr) -> Sum/5
  yaw factors/1(Cnp) -> Sum/4
  beta/1 -> 1-D Lookup Table/2
  alpha/1 -> 1-D Lookup Table/1
  1-D Lookup Table/1 -> Sum/1
  Sign/1 -> Product2/2

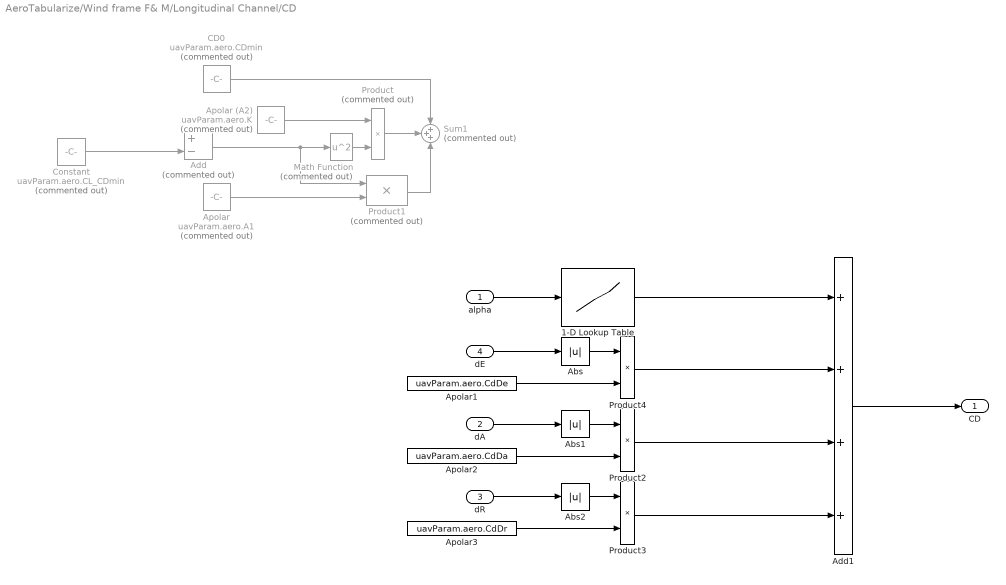
== system AeroTabularize/Wind frame F& M/Longitudinal Channel/CD ==
  alpha : Inport
  dA : Inport  Port=2
  dR : Inport  Port=3
  dE : Inport  Port=4
  1-D Lookup Table : Lookup_n-D  NumberOfTableDimensions=1  BreakpointsForDimension1=uavParam.aero.alpha_lon  Table=uavParam.aero.CD  ExtrapMethod=Clip  UseLastTableValue=on  InternalRulePriority=Speed  RndMeth=Simplest
  Abs : Abs  SaturateOnIntegerOverflow=off
  Abs1 : Abs  SaturateOnIntegerOverflow=off
  Abs2 : Abs  SaturateOnIntegerOverflow=off
  Add : Sum  Commented=on  Inputs=+-
  Add1 : Sum  Inputs=++++
  Apolar : Constant  Commented=on  Value=uavParam.aero.A1
      settings: AttributesFormatString=%<Value>
  Apolar (A2) : Constant  Commented=on  Value=uavParam.aero.K
      settings: AttributesFormatString=%<Value>
  Apolar1 : Constant  Value=uavParam.aero.CdDe
      settings: AttributesFormatString=%<Value>
  Apolar2 : Constant  Value=uavParam.aero.CdDa
      settings: AttributesFormatString=%<Value>
  Apolar3 : Constant  Value=uavParam.aero.CdDr
      settings: AttributesFormatString=%<Value>
  CD0 : Constant  Commented=on  Value=uavParam.aero.CDmin
      settings: AttributesFormatString=%<Value>
  Constant : Constant  Commented=on  Value=uavParam.aero.CL_CDmin
  Math Function : Math  Commented=on  Operator=square  SignedPower=on
  Product : Product  Commented=on  SaturateOnIntegerOverflow=on  OutDataTypeStr=Inherit: Same as first input
  Product1 : Product  Commented=on  SaturateOnIntegerOverflow=on  OutDataTypeStr=Inherit: Same as first input
  Product2 : Product  SaturateOnIntegerOverflow=on  OutDataTypeStr=Inherit: Same as first input
  Product3 : Product  SaturateOnIntegerOverflow=on  OutDataTypeStr=Inherit: Same as first input
  Product4 : Product  SaturateOnIntegerOverflow=on  OutDataTypeStr=Inherit: Same as first input
  Sum1 : Sum  Commented=on  Inputs=+++  SaturateOnIntegerOverflow=on
  CD : Outport  VectorParamsAs1DForOutWhenUnconnected=off
  wires:
  Add1/1 -> CD/1
  Apolar (A2)/1 -> Product/1
  Math Function/1 -> Product/2
  Product1/1 -> Sum1/3
  Product/1 -> Sum1/2
  Add/1 -> Product1/1, Math Function/1
  CD0/1 -> Sum1/1
  Apolar/1 -> Product1/2
  Constant/1 -> Add/2
  Apolar1/1 -> Product4/2
  dE/1 -> Abs/1
  Abs/1 -> Product4/1
  Abs1/1 -> Product2/1
  Apolar2/1 -> Product2/2
  dA/1 -> Abs1/1
  Abs2/1 -> Product3/1
  Apolar3/1 -> Product3/2
  dR/1 -> Abs2/1
  Product4/1 -> Add1/2
  Product2/1 -> Add1/3
  Product3/1 -> Add1/4
  alpha/1 -> 1-D Lookup Table/1
  1-D Lookup Table/1 -> Add1/1

== system AeroTabularize/Wind frame F& M/Longitudinal Channel/CL ==
  alpha : Inport
  alpha_dot : Inport  Port=2
  dE : Inport  Port=3
  p,q,r : Inport  Port=4
  Airspeed : Inport  Port=5
  dA : Inport  Port=6
  1-D Lookup Table : Lookup_n-D  NumberOfTableDimensions=1  BreakpointsForDimension1=uavParam.aero.alpha_lon  Table=uavParam.aero.CL  ExtrapMethod=Clip  UseLastTableValue=on  InternalRulePriority=Speed  RndMeth=Simplest
  Abs : Abs  SaturateOnIntegerOverflow=off
  CL1 : Constant  Value=uavParam.aero.CLDa
      settings: AttributesFormatString=%<Value>
  CLDe : Constant  Value=uavParam.aero.CLDe
      settings: AttributesFormatString=%<Value>
  CLa_dot : Constant  Value=uavParam.aero.CLa_dot
      settings: AttributesFormatString=%<Value>
  Lift due to pitch rate : Subsystem
  Product1 : Product  SaturateOnIntegerOverflow=on  OutDataTypeStr=Inherit: Same as first input
  Product2 : Product  SaturateOnIntegerOverflow=on  OutDataTypeStr=Inherit: Same as first input
  Product5 : Product  SaturateOnIntegerOverflow=on  OutDataTypeStr=Inherit: Same as first input
  Sum : Sum  Inputs=+++++  SaturateOnIntegerOverflow=on
  CL : Outport  VectorParamsAs1DForOutWhenUnconnected=off
  wires:
  Airspeed/1 -> Lift due to pitch rate/2(Airspeed)
  p,q,r/1 -> Lift due to pitch rate/1(p,q,r)
  Sum/1 -> CL/1
  dE/1 -> Product1/2
  CLDe/1 -> Product1/1
  alpha_dot/1 -> Product5/2
  CLa_dot/1 -> Product5/1
  CL1/1 -> Product2/2
  dA/1 -> Abs/1
  Abs/1 -> Product2/1
  alpha/1 -> 1-D Lookup Table/1
  1-D Lookup Table/1 -> Sum/1
  Product5/1 -> Sum/2
  Lift due to pitch rate/1(CLq) -> Sum/5
  Product1/1 -> Sum/3
  Product2/1 -> Sum/4

== system AeroTabularize/Wind frame F& M/Longitudinal Channel/Cm ==
  alpha : Inport
  dE : Inport  Port=2
  p,q,r : Inport  Port=3
  Airspeed : Inport  Port=4
  1-D Lookup Table : Lookup_n-D  NumberOfTableDimensions=1  BreakpointsForDimension1=uavParam.aero.alpha_lon  Table=uavParam.aero.CM  ExtrapMethod=Clip  UseLastTableValue=on  InternalRulePriority=Speed  RndMeth=Simplest
  CmDe : Constant  Value=uavParam.aero.CmDe
      settings: AttributesFormatString=%<Value>
  Lift due to pitch rate : Subsystem
  Product1 : Product  Inputs=**  SaturateOnIntegerOverflow=on  OutDataTypeStr=Inherit: Same as first input
  Sum : Sum  Inputs=+++  SaturateOnIntegerOverflow=on
  Cm : Outport  VectorParamsAs1DForOutWhenUnconnected=off
  wires:
  Lift due to pitch rate/1(Cmq) -> Sum/3  "cmq"
  p,q,r/1 -> Lift due to pitch rate/1(p,q,r)
  1-D Lookup Table/1 -> Sum/1  "cma"
  Sum/1 -> Cm/1  "total"
  dE/1 -> Product1/2
  CmDe/1 -> Product1/1
  Airspeed/1 -> Lift due to pitch rate/2(Airspeed)
  alpha/1 -> 1-D Lookup Table/1
  Product1/1 -> Sum/2  "cmde"

== system AeroTabularize/Wind frame F& M1/Lateral Channel/CY ==
  beta : Inport
  dR : Inport  Port=2
  p,q,r : Inport  Port=3
  Airspeed : Inport  Port=4
  1-D Lookup Table : Lookup_n-D  NumberOfTableDimensions=1  BreakpointsForDimension1=uavParam.aero.beta  Table=uavParam.aero.CY  ExtrapMethod=Clip  UseLastTableValue=on  InternalRulePriority=Speed  RndMeth=Simplest
  Abs : Abs  SaturateOnIntegerOverflow=off
  CYDr : Constant  Value=uavParam.aero.CYDr
      settings: AttributesFormatString=%<Value>
  CYb : Constant  Commented=on  Value=uavParam.aero.CYb
      settings: AttributesFormatString=%<Value>
  Product : Product  Commented=on  SaturateOnIntegerOverflow=on  OutDataTypeStr=Inherit: Same as first input
  Product1 : Product  SaturateOnIntegerOverflow=on  OutDataTypeStr=Inherit: Same as first input
  Product2 : Product
  Sign : Signum
  Sum2 : Sum  Inputs=++++  SaturateOnIntegerOverflow=on
  roll factors : Subsystem
  CY : Outport  VectorParamsAs1DForOutWhenUnconnected=off
  wires:
  Product1/1 -> Sum2/2
  dR/1 -> Product1/2
  CYDr/1 -> Product1/1
  CYb/1 -> Product/1
  Airspeed/1 -> roll factors/2(Airspeed)
  p,q,r/1 -> roll factors/1(p,q,r)
  roll factors/1(CYp) -> Sum2/3
  roll factors/2(CYr) -> Sum2/4
  Sum2/1 -> CY/1
  beta/1 -> Sign/1, Abs/1
  Abs/1 -> 1-D Lookup Table/1
  Product2/1 -> Sum2/1
  1-D Lookup Table/1 -> Product2/1
  Sign/1 -> Product2/2

== system AeroTabularize/Wind frame F& M1/Lateral Channel/Cl ==
  beta : Inport
  dA : Inport  Port=2
  dR : Inport  Port=3
  p,q,r : Inport  Port=4
  Airspeed : Inport  Port=5
  1-D Lookup Table : Lookup_n-D  NumberOfTableDimensions=1  BreakpointsForDimension1=uavParam.aero.beta  Table=uavParam.aero.CR  InternalRulePriority=Speed  RndMeth=Simplest
  Abs : Abs  SaturateOnIntegerOverflow=off
  ClDa : Constant  Value=uavParam.aero.ClDa
      settings: AttributesFormatString=%<Value>
  ClDr : Constant  Value=uavParam.aero.ClDr
      settings: AttributesFormatString=%<Value>
  Clb : Constant  Commented=on  Value=uavParam.aero.Clb
      settings: AttributesFormatString=%<Value>
  Gain4 : Gain  Gain=-1
  Product1 : Product  SaturateOnIntegerOverflow=on  OutDataTypeStr=Inherit: Same as first input
  Product2 : Product
  Product5 : Product  SaturateOnIntegerOverflow=on  OutDataTypeStr=Inherit: Same as first input
  Sign : Signum
  Sum : Sum  Inputs=+++++  SaturateOnIntegerOverflow=on
  roll factors : Subsystem
  Cl : Outport  VectorParamsAs1DForOutWhenUnconnected=off
  wires:
  roll factors/1(Clp) -> Sum/4
  Product5/1 -> Sum/2  "CldA"
  Airspeed/1 -> roll factors/2(Airspeed)
  p,q,r/1 -> roll factors/1(p,q,r)
  roll factors/2(Clr) -> Sum/5
  Product1/1 -> Sum/3  "Cldr"
  Sum/1 -> Cl/1
  dR/1 -> Product1/2
  ClDr/1 -> Product1/1
  dA/1 -> Product5/2
  ClDa/1 -> Product5/1
  Clb/1 -> ?
  Product2/1 -> Gain4/1
  Sign/1 -> Product2/2
  beta/1 -> Sign/1, Abs/1
  Abs/1 -> 1-D Lookup Table/1
  1-D Lookup Table/1 -> Product2/1  "Clb"
  Gain4/1 -> Sum/1

== system AeroTabularize/Wind frame F& M1/Lateral Channel/Cn ==
  beta : Inport
  dA : Inport  Port=2
  dR : Inport  Port=3
  p,q,r : Inport  Port=4
  Airspeed : Inport  Port=5
  1-D Lookup Table : Lookup_n-D  NumberOfTableDimensions=1  BreakpointsForDimension1=uavParam.aero.beta  Table=uavParam.aero.CN  ExtrapMethod=Clip  UseLastTableValue=on  InternalRulePriority=Speed  RndMeth=Simplest
  Abs : Abs  SaturateOnIntegerOverflow=off
  CnDa : Constant  Value=uavParam.aero.CnDa
      settings: AttributesFormatString=%<Value>
  CnDr : Constant  Value=uavParam.aero.CnDr
      settings: AttributesFormatString=%<Value>
  Cnb : Constant  Commented=on  Value=uavParam.aero.Cnb
      settings: AttributesFormatString=%<Value>
  Gain : Gain  Gain=-1
  Product1 : Product  SaturateOnIntegerOverflow=on  OutDataTypeStr=Inherit: Same as first input
  Product2 : Product
  Product5 : Product  SaturateOnIntegerOverflow=on  OutDataTypeStr=Inherit: Same as first input
  Sign : Signum
  Sum : Sum  Inputs=+++++  SaturateOnIntegerOverflow=on
  yaw factors : Subsystem
  Cn : Outport  VectorParamsAs1DForOutWhenUnconnected=off
  wires:
  Airspeed/1 -> yaw factors/2(Airspeed)
  p,q,r/1 -> yaw factors/1(p,q,r)
  CnDa/1 -> Product5/1
  Product5/1 -> Sum/2
  dA/1 -> Product5/2
  CnDr/1 -> Product1/1
  dR/1 -> Product1/2
  Sum/1 -> Cn/1
  Product1/1 -> Sum/3
  yaw factors/2(Cnr) -> Sum/5
  yaw factors/1(Cnp) -> Sum/4
  beta/1 -> Sign/1, Abs/1
  Abs/1 -> 1-D Lookup Table/1
  1-D Lookup Table/1 -> Product2/1
  Sign/1 -> Product2/2
  Product2/1 -> Gain/1
  Gain/1 -> Sum/1

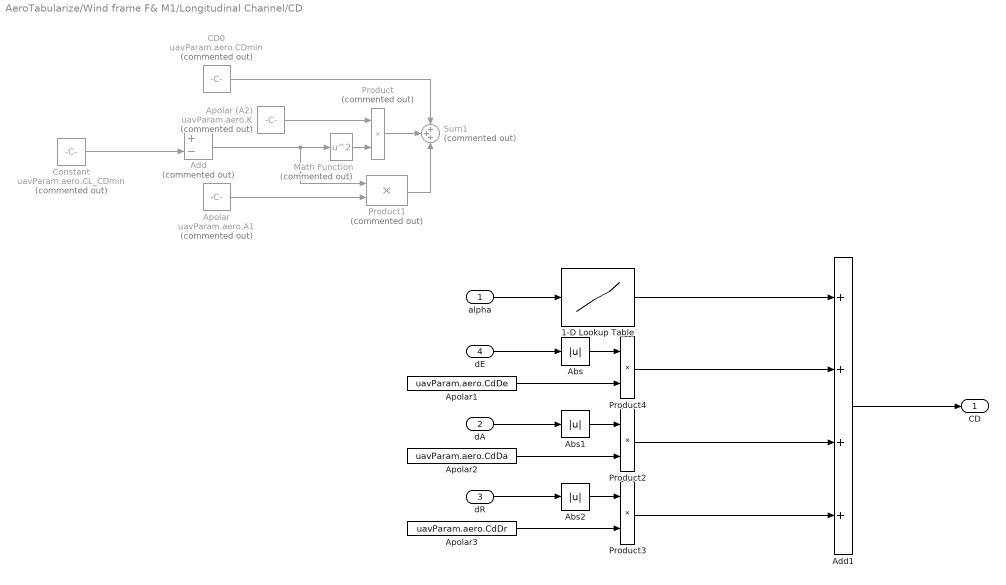
== system AeroTabularize/Wind frame F& M1/Longitudinal Channel/CD ==
  alpha : Inport
  dA : Inport  Port=2
  dR : Inport  Port=3
  dE : Inport  Port=4
  1-D Lookup Table : Lookup_n-D  NumberOfTableDimensions=1  BreakpointsForDimension1=uavParam.aero.alpha  Table=uavParam.aero.CD  ExtrapMethod=Clip  UseLastTableValue=on  InternalRulePriority=Speed  RndMeth=Simplest
  Abs : Abs  SaturateOnIntegerOverflow=off
  Abs1 : Abs  SaturateOnIntegerOverflow=off
  Abs2 : Abs  SaturateOnIntegerOverflow=off
  Add : Sum  Commented=on  Inputs=+-
  Add1 : Sum  Inputs=++++
  Apolar : Constant  Commented=on  Value=uavParam.aero.A1
      settings: AttributesFormatString=%<Value>
  Apolar (A2) : Constant  Commented=on  Value=uavParam.aero.K
      settings: AttributesFormatString=%<Value>
  Apolar1 : Constant  Value=uavParam.aero.CdDe
      settings: AttributesFormatString=%<Value>
  Apolar2 : Constant  Value=uavParam.aero.CdDa
      settings: AttributesFormatString=%<Value>
  Apolar3 : Constant  Value=uavParam.aero.CdDr
      settings: AttributesFormatString=%<Value>
  CD0 : Constant  Commented=on  Value=uavParam.aero.CDmin
      settings: AttributesFormatString=%<Value>
  Constant : Constant  Commented=on  Value=uavParam.aero.CL_CDmin
  Math Function : Math  Commented=on  Operator=square  SignedPower=on
  Product : Product  Commented=on  SaturateOnIntegerOverflow=on  OutDataTypeStr=Inherit: Same as first input
  Product1 : Product  Commented=on  SaturateOnIntegerOverflow=on  OutDataTypeStr=Inherit: Same as first input
  Product2 : Product  SaturateOnIntegerOverflow=on  OutDataTypeStr=Inherit: Same as first input
  Product3 : Product  SaturateOnIntegerOverflow=on  OutDataTypeStr=Inherit: Same as first input
  Product4 : Product  SaturateOnIntegerOverflow=on  OutDataTypeStr=Inherit: Same as first input
  Sum1 : Sum  Commented=on  Inputs=+++  SaturateOnIntegerOverflow=on
  CD : Outport  VectorParamsAs1DForOutWhenUnconnected=off
  wires:
  Add1/1 -> CD/1
  Apolar (A2)/1 -> Product/1
  Math Function/1 -> Product/2
  Product1/1 -> Sum1/3
  Product/1 -> Sum1/2
  Add/1 -> Product1/1, Math Function/1
  CD0/1 -> Sum1/1
  Apolar/1 -> Product1/2
  Constant/1 -> Add/2
  Apolar1/1 -> Product4/2
  dE/1 -> Abs/1
  Abs/1 -> Product4/1
  Abs1/1 -> Product2/1
  Apolar2/1 -> Product2/2
  dA/1 -> Abs1/1
  Abs2/1 -> Product3/1
  Apolar3/1 -> Product3/2
  dR/1 -> Abs2/1
  Product4/1 -> Add1/2
  Product2/1 -> Add1/3
  Product3/1 -> Add1/4
  alpha/1 -> 1-D Lookup Table/1
  1-D Lookup Table/1 -> Add1/1

== system AeroTabularize/Wind frame F& M1/Longitudinal Channel/CL ==
  alpha : Inport
  alpha_dot : Inport  Port=2
  dE : Inport  Port=3
  p,q,r : Inport  Port=4
  Airspeed : Inport  Port=5
  dA : Inport  Port=6
  1-D Lookup Table : Lookup_n-D  NumberOfTableDimensions=1  BreakpointsForDimension1=uavParam.aero.alpha  Table=uavParam.aero.CL  ExtrapMethod=Clip  UseLastTableValue=on  InternalRulePriority=Speed  RndMeth=Simplest
  Abs : Abs  SaturateOnIntegerOverflow=off
  CL1 : Constant  Value=uavParam.aero.CLDa
      settings: AttributesFormatString=%<Value>
  CLDe : Constant  Value=uavParam.aero.CLDe
      settings: AttributesFormatString=%<Value>
  CLa_dot : Constant  Value=uavParam.aero.CLa_dot
      settings: AttributesFormatString=%<Value>
  Lift due to pitch rate : Subsystem
  Product1 : Product  SaturateOnIntegerOverflow=on  OutDataTypeStr=Inherit: Same as first input
  Product2 : Product  SaturateOnIntegerOverflow=on  OutDataTypeStr=Inherit: Same as first input
  Product5 : Product  SaturateOnIntegerOverflow=on  OutDataTypeStr=Inherit: Same as first input
  Sum : Sum  Inputs=+++++  SaturateOnIntegerOverflow=on
  CL : Outport  VectorParamsAs1DForOutWhenUnconnected=off
  wires:
  Airspeed/1 -> Lift due to pitch rate/2(Airspeed)
  p,q,r/1 -> Lift due to pitch rate/1(p,q,r)
  Sum/1 -> CL/1
  dE/1 -> Product1/2
  CLDe/1 -> Product1/1
  alpha_dot/1 -> Product5/2
  CLa_dot/1 -> Product5/1
  CL1/1 -> Product2/2
  dA/1 -> Abs/1
  Abs/1 -> Product2/1
  alpha/1 -> 1-D Lookup Table/1
  1-D Lookup Table/1 -> Sum/1
  Product5/1 -> Sum/2
  Lift due to pitch rate/1(CLq) -> Sum/5
  Product1/1 -> Sum/3
  Product2/1 -> Sum/4

== system AeroTabularize/Wind frame F& M1/Longitudinal Channel/Cm ==
  alpha : Inport
  dE : Inport  Port=2
  p,q,r : Inport  Port=3
  Airspeed : Inport  Port=4
  1-D Lookup Table : Lookup_n-D  NumberOfTableDimensions=1  BreakpointsForDimension1=uavParam.aero.alpha  Table=uavParam.aero.CM  ExtrapMethod=Clip  UseLastTableValue=on  InternalRulePriority=Speed  RndMeth=Simplest
  CmDe : Constant  Value=uavParam.aero.CmDe
      settings: AttributesFormatString=%<Value>
  Lift due to pitch rate : Subsystem
  Product1 : Product  Inputs=**  SaturateOnIntegerOverflow=on  OutDataTypeStr=Inherit: Same as first input
  Sum : Sum  Inputs=+++  SaturateOnIntegerOverflow=on
  Cm : Outport  VectorParamsAs1DForOutWhenUnconnected=off
  wires:
  Lift due to pitch rate/1(Cmq) -> Sum/3  "cmq"
  p,q,r/1 -> Lift due to pitch rate/1(p,q,r)
  1-D Lookup Table/1 -> Sum/1  "cma"
  Sum/1 -> Cm/1  "total"
  dE/1 -> Product1/2
  CmDe/1 -> Product1/1
  Airspeed/1 -> Lift due to pitch rate/2(Airspeed)
  alpha/1 -> 1-D Lookup Table/1
  Product1/1 -> Sum/2  "cmde"
